simulink model "ppsim"  (R2024b)
settings: Solver=VariableStepAuto  StartTime=0.0  StopTime=20  RelTol=1e-3
values from neighbouring files (symbols this model uses):
  dtflin = dtftust(tflin, Ts)    [disc.m]    (also in main.m)
  PpReg = ppc(dtflin, [0.01 0.1 0.1 0.1])    [main.m]
  z = -0.1    [main.m]
settings Model: Creator=markminerov  LastModifiedBy=markminerov
settings DebuggingCC: AlgebraicLoopMsg=none

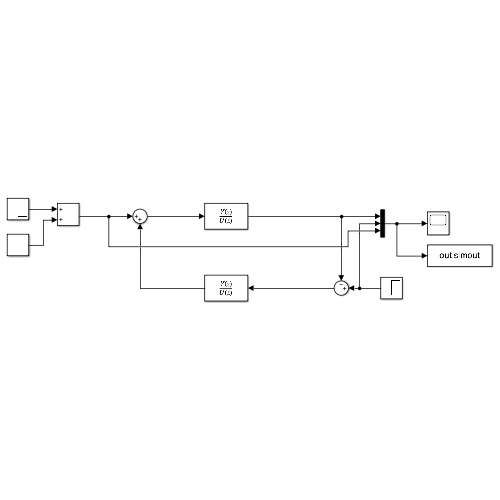
[thumbnail: Simulink's stored preview of the top-level diagram]
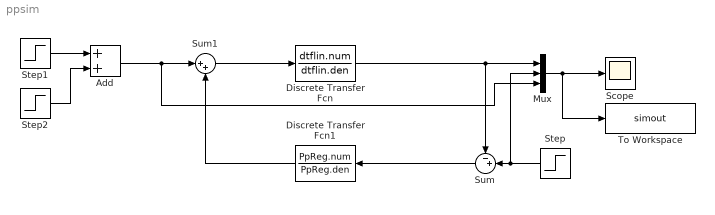
== system ppsim ==
  Add : Sum
  Discrete Transfer Fcn : DiscreteTransferFcn  Numerator=dtflin.num  Denominator=dtflin.den
  Discrete Transfer Fcn1 : DiscreteTransferFcn  Numerator=PpReg.num  Denominator=PpReg.den
  Mux : Mux  Inputs=3
  Scope : Scope
  Step : Step  After=u  SampleTime=0
  Step1 : Step  Time=11  After=z  SampleTime=0
  Step2 : Step  Time=12  After=-z  SampleTime=0
  Sum : Sum  Inputs=-+|
  Sum1 : Sum  Inputs=|++
  To Workspace : ToWorkspace  VariableName=simout  SaveFormat=Timeseries  SampleTime=-1
  wires:
  Discrete Transfer Fcn/1 -> Mux/1, Sum/1
  Step/1 -> Mux/2, Sum/2
  Sum/1 -> Discrete Transfer Fcn1/1
  Step1/1 -> Add/1
  Step2/1 -> Add/2
  Add/1 -> Mux/3, Sum1/1
  Sum1/1 -> Discrete Transfer Fcn/1
  Discrete Transfer Fcn1/1 -> Sum1/2
  Mux/1 -> To Workspace/1, Scope/1
